simulink model "xiti4_12"  (Simulink 5.0)
settings: Solver=ode45  StartTime=0.0  StopTime=100  RelTol=1e-3
libraries: simulink_extras x2
settings Model: LastModifiedBy=ThinkPad  ExtModeTrigMode=oneshot  ExtModeArmWhenConnect=off  LimitDataPoints=off  BooleanDataType=off

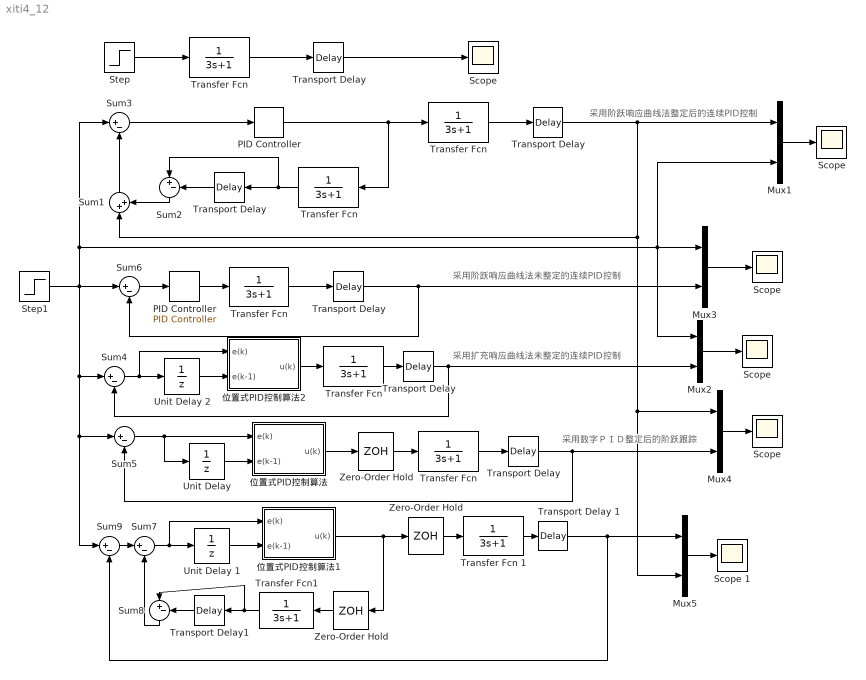
== system xiti4_12 ==
  note: 采用阶跃响应曲线法整定后的连续PID控制
  note: 采用阶跃响应曲线法未整定的连续PID控制
  note: 采用扩充响应曲线法未整定的连续PID控制
  note: 采用数字ＰＩＤ整定后的阶跃跟踪
  "   Scope   " : Scope
      settings: YMin=-3.5  YMax=1  MaxDataPoints=500000
  "  Transfer Fcn " : TransferFcn  Denominator=[3 1]
  "  Transfer Fcn   " : TransferFcn  Denominator=[3 1]
  " PID Controller " : simulink_extras/Additional Linear/PID Controller  P=2.4  I=0.533  D=1.8
  " Scope" : Scope
      settings: YMin=0  YMax=110  MaxDataPoints=500000
  " Scope " : Scope
      settings: YMin=-3.5  YMax=1  SaveName=ScopeData2  MaxDataPoints=500000
  " Scope 1" : Scope
      settings: YMin=-3.5  YMax=1  SaveName=ScopeData4  MaxDataPoints=500000
  " Transfer Fcn " : TransferFcn  Denominator=[3 1]
  " Transport Delay" : TransportDelay  DelayTime=1.5
  Mux{1..5} (5 alike) : Mux  Inputs=2
  PID Controller : simulink_extras/Additional Linear/PID Controller  P=0.6  I=0.4/3  D=0.45
  Scope : Scope
      settings: YMin=0  YMax=110  SaveName=ScopeData3  MaxDataPoints=500000
  "Scope " : Scope
      settings: YMin=0  YMax=80  SaveName=S1  DataFormat=Array  MaxDataPoints=500000
  Step : Step  Time=0  SampleTime=0
  Step1 : Step  Time=0  SampleTime=0
  Sum1 : Sum  Orientation=up  Inputs=|++  SaturateOnIntegerOverflow=on
  Sum2 : Sum  Orientation=down  Inputs=|+-  SaturateOnIntegerOverflow=on
  Sum{3..7,9} (6 alike) : Sum  Inputs=|+-  SaturateOnIntegerOverflow=on
  Sum8 : Sum  Orientation=down  Inputs=|+-  SaturateOnIntegerOverflow=on
  Transfer Fcn : TransferFcn  Orientation=left  Denominator=[3 1]
  "Transfer Fcn " : TransferFcn  Denominator=[3 1]
  "Transfer Fcn  " : TransferFcn  Denominator=[3 1]
  Transfer Fcn 1 : TransferFcn  Denominator=[3 1]
  Transfer Fcn1 : TransferFcn  Orientation=left  Denominator=[3 1]
  Transport Delay : TransportDelay  Orientation=left  DelayTime=1.5
  "Transport Delay " : TransportDelay  DelayTime=1.5
  "Transport Delay   " : TransportDelay  DelayTime=1.5
  "Transport Delay    " : TransportDelay  DelayTime=1.5
  "Transport Delay     " : TransportDelay  DelayTime=1.5
  Transport Delay 1 : TransportDelay  DelayTime=1.5
  Transport Delay1 : TransportDelay  Orientation=left  DelayTime=1.5
  "Unit Delay " : UnitDelay  SampleTime=0.25
  Unit Delay 1 : UnitDelay  SampleTime=0.25
  Unit Delay 2 : UnitDelay  SampleTime=0.25
  Zero-Order Hold : ZeroOrderHold  Orientation=left  SampleTime=0.25
  "Zero-Order Hold " : ZeroOrderHold  SampleTime=0.25
  "Zero-Order Hold   " : ZeroOrderHold  SampleTime=0.25
  位置式PID控制算法 : Subsystem
  位置式PID控制算法1 : Subsystem
  位置式PID控制算法2 : Subsystem
  wires:
  "Transfer Fcn "/1 -> "Transport Delay "/1
  Step1/1 -> Sum6/1, Sum3/1, Mux1/2, Mux3/1, Mux2/1, Sum4/1, Sum5/1, Sum9/1
  " Transfer Fcn "/1 -> " Transport Delay"/1
  " Transport Delay"/1 -> Sum6/2, Mux3/2
  " PID Controller "/1 -> " Transfer Fcn "/1
  Sum6/1 -> " PID Controller "/1
  Mux3/1 -> Scope/1
  "Transfer Fcn  "/1 -> "Transport Delay   "/1
  "Transport Delay   "/1 -> Mux1/1, Sum1/1, Mux4/1, Mux5/2
  Sum3/1 -> PID Controller/1
  Transfer Fcn/1 -> Sum2/1, Transport Delay/1
  Transport Delay/1 -> Sum2/2
  Sum1/1 -> Sum3/2
  Mux1/1 -> "   Scope   "/1
  Sum2/1 -> Sum1/2
  Step/1 -> "Transfer Fcn "/1
  "Transport Delay "/1 -> "Scope "/1
  PID Controller/1 -> "Transfer Fcn  "/1, Transfer Fcn/1
  "  Transfer Fcn "/1 -> "Transport Delay    "/1
  "Transport Delay    "/1 -> Sum4/2, Mux2/2
  位置式PID控制算法2/1(u(k)) -> "  Transfer Fcn "/1
  Mux2/1 -> " Scope"/1
  Mux4/1 -> " Scope "/1
  "Transport Delay     "/1 -> Sum5/2, Mux4/2
  "Unit Delay "/1 -> 位置式PID控制算法/2(e(k-1))
  Sum5/1 -> "Unit Delay "/1, 位置式PID控制算法/1(e(k))
  位置式PID控制算法/1(u(k)) -> "Zero-Order Hold   "/1
  "Zero-Order Hold   "/1 -> "  Transfer Fcn   "/1
  "  Transfer Fcn   "/1 -> "Transport Delay     "/1
  Transfer Fcn 1/1 -> Transport Delay 1/1
  位置式PID控制算法1/1(u(k)) -> "Zero-Order Hold "/1, Zero-Order Hold/1
  Sum9/1 -> Sum7/1
  Transfer Fcn1/1 -> Sum8/1, Transport Delay1/1
  Transport Delay1/1 -> Sum8/2
  Sum8/1 -> Sum7/2
  Zero-Order Hold/1 -> Transfer Fcn1/1
  "Zero-Order Hold "/1 -> Transfer Fcn 1/1
  Mux5/1 -> " Scope 1"/1
  Transport Delay 1/1 -> Mux5/1, Sum9/2
  Unit Delay 1/1 -> 位置式PID控制算法1/2(e(k-1))
  Sum7/1 -> Unit Delay 1/1, 位置式PID控制算法1/1(e(k))
  Sum4/1 -> Unit Delay 2/1, 位置式PID控制算法2/1(e(k))
  Unit Delay 2/1 -> 位置式PID控制算法2/2(e(k-1))

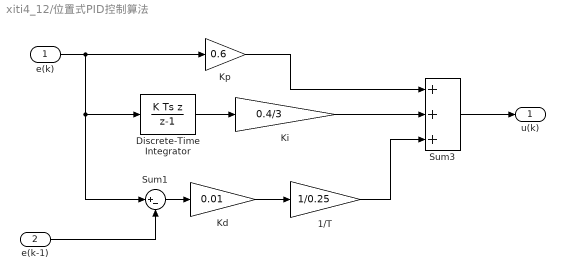
== system xiti4_12/位置式PID控制算法 ==
  e(k) : Inport
  e(k-1) : Inport  Port=2
  1/T : Gain  Gain=1/0.25  SaturateOnIntegerOverflow=on
  Discrete-Time Integrator : DiscreteIntegrator  IntegratorMethod=Backward Euler  SampleTime=0.25
  Kd : Gain  Gain=0.01  SaturateOnIntegerOverflow=on
  Ki : Gain  Gain=0.4/3  SaturateOnIntegerOverflow=on
  Kp : Gain  Gain=0.6  SaturateOnIntegerOverflow=on
  Sum1 : Sum  Inputs=|+-  SaturateOnIntegerOverflow=on
  Sum3 : Sum  Inputs=+++  SaturateOnIntegerOverflow=on
  u(k) : Outport
  wires:
  Discrete-Time Integrator/1 -> Ki/1
  Sum1/1 -> Kd/1
  e(k)/1 -> Kp/1, Discrete-Time Integrator/1, Sum1/1
  Kp/1 -> Sum3/1
  Ki/1 -> Sum3/2
  Sum3/1 -> u(k)/1
  Kd/1 -> 1/T/1
  1/T/1 -> Sum3/3
  e(k-1)/1 -> Sum1/2

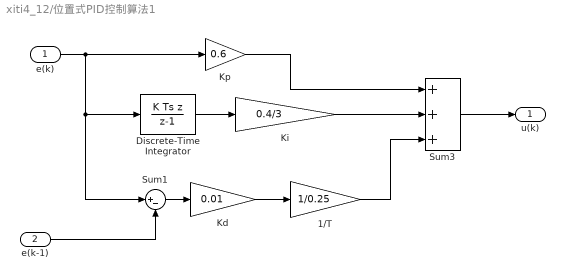
== system xiti4_12/位置式PID控制算法1 ==
  e(k) : Inport
  e(k-1) : Inport  Port=2
  1/T : Gain  Gain=1/0.25  SaturateOnIntegerOverflow=on
  Discrete-Time Integrator : DiscreteIntegrator  IntegratorMethod=Backward Euler  SampleTime=0.25
  Kd : Gain  Gain=0.01  SaturateOnIntegerOverflow=on
  Ki : Gain  Gain=0.4/3  SaturateOnIntegerOverflow=on
  Kp : Gain  Gain=0.6  SaturateOnIntegerOverflow=on
  Sum1 : Sum  Inputs=|+-  SaturateOnIntegerOverflow=on
  Sum3 : Sum  Inputs=+++  SaturateOnIntegerOverflow=on
  u(k) : Outport
  wires:
  e(k-1)/1 -> Sum1/2
  1/T/1 -> Sum3/3
  Kd/1 -> 1/T/1
  Sum3/1 -> u(k)/1
  Ki/1 -> Sum3/2
  Kp/1 -> Sum3/1
  e(k)/1 -> Sum1/1, Discrete-Time Integrator/1, Kp/1
  Sum1/1 -> Kd/1
  Discrete-Time Integrator/1 -> Ki/1

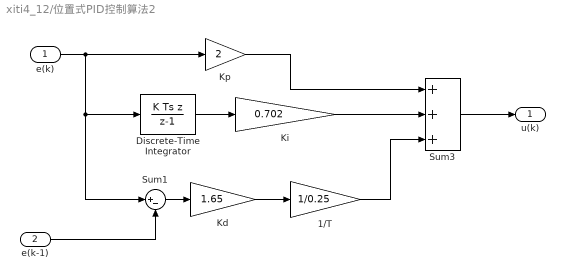
== system xiti4_12/位置式PID控制算法2 ==
  e(k) : Inport
  e(k-1) : Inport  Port=2
  1/T : Gain  Gain=1/0.25  SaturateOnIntegerOverflow=on
  Discrete-Time Integrator : DiscreteIntegrator  IntegratorMethod=Backward Euler  SampleTime=0.25
  Kd : Gain  Gain=1.65  SaturateOnIntegerOverflow=on
  Ki : Gain  Gain=0.702  SaturateOnIntegerOverflow=on
  Kp : Gain  Gain=2  SaturateOnIntegerOverflow=on
  Sum1 : Sum  Inputs=|+-  SaturateOnIntegerOverflow=on
  Sum3 : Sum  Inputs=+++  SaturateOnIntegerOverflow=on
  u(k) : Outport
  wires:
  e(k-1)/1 -> Sum1/2
  1/T/1 -> Sum3/3
  Kd/1 -> 1/T/1
  Sum3/1 -> u(k)/1
  Ki/1 -> Sum3/2
  Kp/1 -> Sum3/1
  e(k)/1 -> Sum1/1, Discrete-Time Integrator/1, Kp/1
  Sum1/1 -> Kd/1
  Discrete-Time Integrator/1 -> Ki/1
